simulink model "X31dynamics_03_controller_MG"  (R2014b)
settings: Solver=ode45  StartTime=0.0  StopTime=10.0  RelTol=1e-3
InitFcn:
  | X31dynamics_03_controller_MG_init
undefined symbols (not defined in the file or in its folder): X31_MnvrGen
libraries: simulink x10
settings Model: Creator=5909  LastModifiedBy=5909
settings OptimizationCC: InlineParams=on

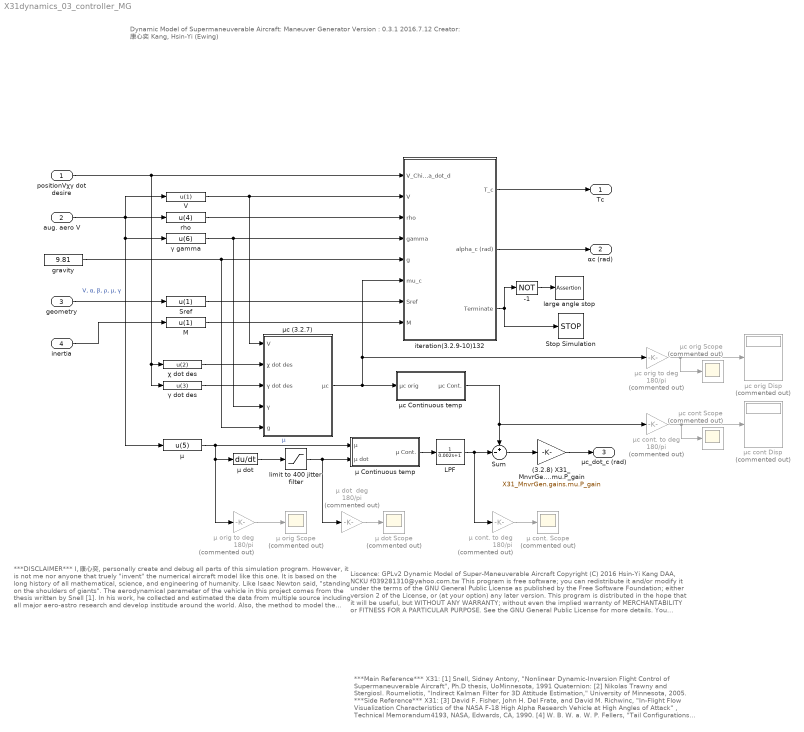
== system X31dynamics_03_controller_MG ==
  note: Dynamic Model of Supermaneuverable Aircraft:
      | Maneuver Generator
      | Version : 0.3.1
      | 2016.7.12
      | Creator: 康心奕 Kang, Hsin-Yi (Ewing)
  note: Liscence: GPLv2
      | Dynamic Model of Super-Maneuverable Aircraft
      | Copyright (C) 2016 Hsin-Yi Kang
      | DAA, NCKU
      | f039281310@yahoo.com.tw
      | This program is free software; you can redistribute it and/or modify it under the terms of the GNU General Public License as published by the Free Software Foundation; either version 2 of the License, or (at your option) any later version. This program is distributed in the hope that it will be useful, but WITHOUT ANY WARRANTY; without even the implied warranty of MERCHANTABILITY or FITNESS FOR A PARTICULAR PURPOSE. See the GNU General Public License for more details. You should have received a copy of the GNU General Public License along with this program; if not, write to the Free Software Foundation, Inc., 51 Franklin Street, Fifth Floor, Boston, MA 02110-1301, USA.
  note: ***DISCLAIMER***
      | I, 康心奕, personally create and debug all parts of this simulation program. However, it is not me nor anyone that truely "invent" the numerical aircraft model like this one. It is based on the long history of all mathematical, science, and engineering of humanity. Like Isaac Newton said, "standing on the shoulders of giants".
      | The aerodynamical parameter of the vehicle in this project comes from the thesis written by Snell [1]. In his work, he collected and estimated the data from multiple source including all major aero-astro research and develop institude around the world. Also, the method to model the dynamics of the vehicle and the controller implemented including the NDI and Gain Scheduling also came from his thesis.
      | The quaternion kinematics mainly reference to the toturial paper done by Trawny [2], where he collected and organized all fundamental properties and mathematical operation of such system.
      | This model is released to improve our ability to understand and develop control methodology of aerial vehicle system similar to this one. It is released free of charge now and always will be so in the hope of sharing the knowledge as much as possible and making this world a better place.
      | However, despite my greatest effort to ensure the correctness of the code, it is not garantee to be free of bug or other issue. You are free to use and modify the program to meet your need but I'm not responsible for any potential risk or damaged of any kind.
      |
      | Long live and prosper
  note: ***Main Reference***
      | X31:
      | [1] Snell, Sidney Antony, "Nonlinear Dynamic-Inversion Flight Control of Supermaneuverable Aircraft", Ph.D thesis, UoMinnesota, 1991
      | Quaternion:
      | [2] Nikolas Trawny and StergiosI. Roumeliotis, "Indirect Kalman Filter for 3D Attitude Estimation," University of Minnesota, 2005.
      |
      | ***Side Reference***
      | X31:
      | [3] David F. Fisher, John H. Del Frate, and David M. Richwinc, "In-Flight Flow Visualization Characteristics of the NASA F-18 High Alpha Research Vehicle at High Angles of Attack"
      | , Technical Memorandum4193, NASA, Edwards, CA, 1990.
      | [4] W. B. W. a. W. P. Fellers, "Tail Configurations for Highly Maneuverable Aircraft," AGARD, 1981.
      |
      | Quaternion:
      | [5] Nikolas Trawnyand StergiosI. Roumeliotis, "Indirect Kalman Filter for 3D Attitude Estimation," University of Minnesota, 2005.
      | [6] W. G. Breckenridge, "Quaternions -Proposed Standard Conventions," JPL, Tech. Rep. INTEROFFICE MEMORANDUM 343-79-1199, 1999.
      | [7] D. M. Henderson, "EularAngles, Quaternions, and Transformation Matrices," Mission Planning and Analysis Division, NASA, July 1977.
  positionVχγ dot desire : Inport  PortDimensions=3
  aug. aero V : Inport  Port=2  PortDimensions=6
  geometry : Inport  Port=3  PortDimensions=7
  inertia : Inport  Port=4  PortDimensions=7
  (3.2.8) X31_MnvrGen.gains.mu.P_gain : Gain  Gain=X31_MnvrGen.gains.mu.P_gain
  -1 : Logic  Operator=NOT  AllPortsSameDT=off  OutDataTypeStr=boolean
  LPF : TransferFcn  Denominator=[0.002 1]
  M : Fcn  Expr=u(1)
  Sref : Fcn  Expr=u(1)
  Stop Simulation : Stop
  Sum : Sum  Inputs=+-|
  V : Fcn  Expr=u(1)
  gravity : Constant  Value=9.81
  iteration(3.2.9-10)132 : Subsystem
  large angle stop : Assertion  AssertionFailFcn=warning('Maneuver Generator fails with large angle')  StopWhenAssertionFail=off
  limit to 400 jitter filter : Saturate  UpperLimit=400  LowerLimit=-400
  rho : Fcn  Expr=u(4)
  γ dot des : Fcn  Expr=u(3)
  γ gamma : Fcn  Expr=u(6)
  μ : Fcn  Expr=u(5)
  μ Continuous temp : Subsystem
  μ cont. Scope : Scope  Commented=on
      settings: YMin=-400  YMax=0  SaveName=ScopeData21
  μ cont. to deg : Gain  Commented=on  Gain=180/pi
  μ dot : Derivative
  μ dot  deg : Gain  Commented=on  Gain=180/pi
  μ dot Scope : Scope  Commented=on
      settings: YMin=-3e+08  YMax=1e+08  SaveName=ScopeData2
  μ orig Scope : Scope  Commented=on
      settings: YMin=-200  YMax=100
  μ orig to deg : Gain  Commented=on  Gain=180/pi
  μc (3.2.7) : Subsystem
  μc Continuous temp : Subsystem
  μc cont Disp : Display  Commented=on
  μc cont Scope : Scope  Commented=on
      settings: TimeRange=3.005065038857998  YMin=-240  YMax=-195
  μc cont. to deg : Gain  Commented=on  Gain=180/pi
  μc orig Disp : Display  Commented=on
  μc orig Scope : Scope  Commented=on
      settings: TimeRange=3.005065038857998  YMin=-200  YMax=200  SaveName=ScopeData14
  μc orig to deg : Gain  Commented=on  Gain=180/pi
  χ dot des : Fcn  Expr=u(2)
  Tc : Outport  PortDimensions=1
  αc (rad) : Outport  Port=2  PortDimensions=1
  μc_dot_c (rad) : Outport  Port=3  PortDimensions=1
  wires:
  positionVχγ dot desire/1 -> γ dot des/1, χ dot des/1, iteration(3.2.9-10)132/1(V_Chi_Gamma_dot_d)
  aug. aero V/1 -> μ/1, γ gamma/1, V/1, rho/1  "V, α, β, ρ, μ, γ"
  Sum/1 -> (3.2.8) X31_MnvrGen.gains.mu.P_gain/1
  (3.2.8) X31_MnvrGen.gains.mu.P_gain/1 -> μc_dot_c (rad)/1
  iteration(3.2.9-10)132/2(alpha_c (rad)) -> αc (rad)/1
  iteration(3.2.9-10)132/1(T_c) -> Tc/1
  geometry/1 -> Sref/1
  inertia/1 -> M/1
  V/1 -> μc (3.2.7)/1(V), iteration(3.2.9-10)132/2(V)
  γ dot des/1 -> μc (3.2.7)/3(γ dot des)
  χ dot des/1 -> μc (3.2.7)/2(χ dot des)
  gravity/1 -> μc (3.2.7)/5(g), iteration(3.2.9-10)132/5(g)
  γ gamma/1 -> μc (3.2.7)/4(γ), iteration(3.2.9-10)132/4(gamma)
  rho/1 -> iteration(3.2.9-10)132/3(rho)
  iteration(3.2.9-10)132/3(Terminate) -> Stop Simulation/1, -1/1
  Sref/1 -> iteration(3.2.9-10)132/7(Sref)
  M/1 -> iteration(3.2.9-10)132/8(M)
  -1/1 -> large angle stop/1
  μ cont. to deg/1 -> μ cont. Scope/1
  μ dot/1 -> limit to 400 jitter filter/1
  μc (3.2.7)/1(μc) -> iteration(3.2.9-10)132/6(mu_c), μc orig to deg/1, μc Continuous temp/1(μc orig)
  μ orig to deg/1 -> μ orig Scope/1
  μ/1 -> μ Continuous temp/1(μ), μ dot/1, μ orig to deg/1  "μ"
  μc orig to deg/1 -> μc orig Disp/1, μc orig Scope/1
  μc Continuous temp/1("μc Cont. ") -> μc cont. to deg/1, Sum/1
  μc cont. to deg/1 -> μc cont Disp/1, μc cont Scope/1
  μ dot  deg/1 -> μ dot Scope/1
  μ Continuous temp/1(μ Cont.) -> LPF/1
  LPF/1 -> Sum/2, μ cont. to deg/1
  limit to 400 jitter filter/1 -> μ Continuous temp/2(μ dot), μ dot  deg/1

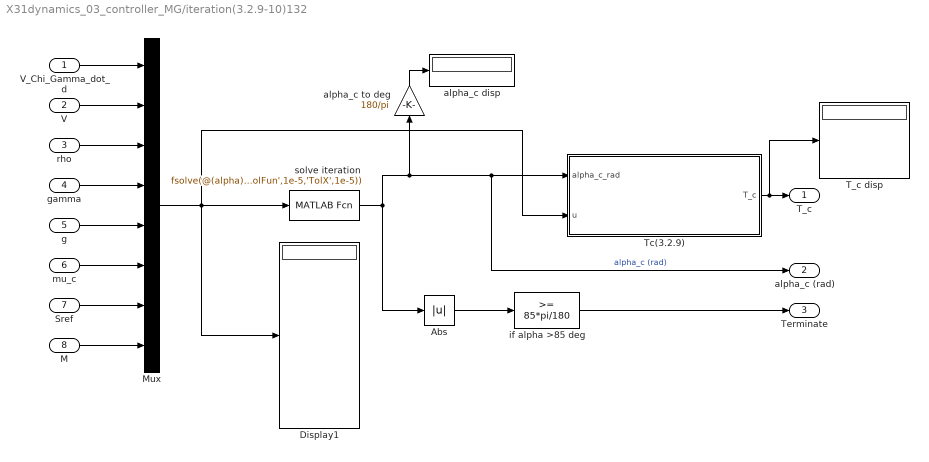
== system X31dynamics_03_controller_MG/iteration(3.2.9-10)132 ==
  V_Chi_Gamma_dot_d : Inport
  V : Inport  Port=2
  rho : Inport  Port=3
  gamma : Inport  Port=4
  g : Inport  Port=5
  mu_c : Inport  Port=6
  Sref : Inport  Port=7
  M : Inport  Port=8
  Abs : Abs
  Display1 : Display
  Mux : Mux  Inputs=8
  T_c disp : Display
  Tc(3.2.9) : MATLAB Function  TreatAsAtomicUnit=on
  alpha_c disp : Display
  alpha_c to deg : Gain  Gain=180/pi
  if alpha >85 deg : simulink/Logic and Bit Operations/Compare To Constant  relop=>=  const=85*pi/180  OutDataTypeStr=boolean
  solve iteration : MATLABFcn  MATLABFcn="fsolve(@(alpha)X31dynamics_03_controller_MG_iter_3_2_9_10(alpha, u(1),u(2), u(3), u(4), u(5),u(6), u(7), u(8), u(9), u(10) ),  10*pi/180, optimset('Display','off', 'TolFun',1e-5,'TolX',1e-5))"
  T_c : Outport
  alpha_c (rad) : Outport  Port=2
  Terminate : Outport  Port=3
  wires:
  V_Chi_Gamma_dot_d/1 -> Mux/1
  V/1 -> Mux/2
  rho/1 -> Mux/3
  gamma/1 -> Mux/4
  g/1 -> Mux/5
  mu_c/1 -> Mux/6
  Sref/1 -> Mux/7
  M/1 -> Mux/8
  Mux/1 -> Display1/1, solve iteration/1, Tc(3.2.9)/2(u)
  solve iteration/1 -> alpha_c (rad)/1, Tc(3.2.9)/1(alpha_c_rad), alpha_c to deg/1, Abs/1  "alpha_c (rad)"
  if alpha >85 deg/1 -> Terminate/1
  Tc(3.2.9)/1(T_c) -> T_c disp/1, T_c/1
  Abs/1 -> if alpha >85 deg/1
  alpha_c to deg/1 -> alpha_c disp/1

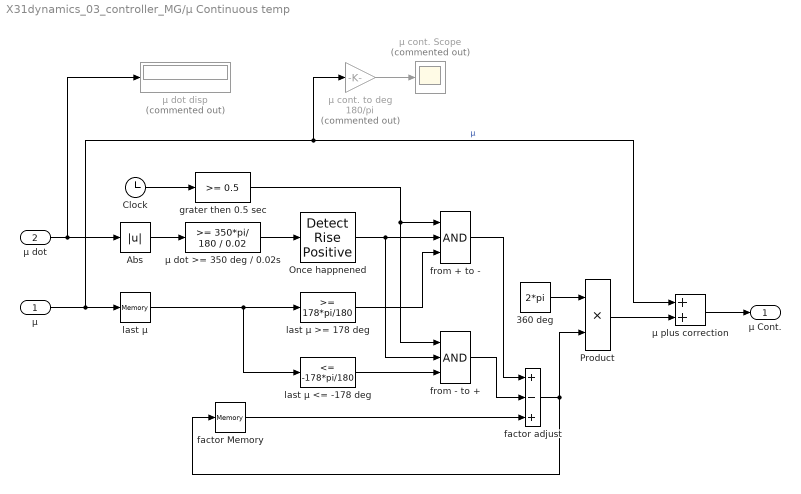
== system X31dynamics_03_controller_MG/μ Continuous temp ==
  μ : Inport
  μ dot : Inport  Port=2
  360 deg : Constant  Value=2*pi
  Abs : Abs
  Clock : Clock
  Once happnened : simulink/Logic and Bit Operations/Detect Rise Positive  vinit=0  InputProcessing=Inherited  OutDataTypeStr=boolean
  Product : Product
  factor Memory : Memory
  factor adjust : Sum  Inputs=+-+
  from + to - : Logic  Inputs=3  AllPortsSameDT=off  OutDataTypeStr=fixdt(1,16)
  from - to + : Logic  Inputs=3  AllPortsSameDT=off  OutDataTypeStr=fixdt(1,16)
  grater then 0.5 sec : simulink/Logic and Bit Operations/Compare To Constant  relop=>=  const=0.5  OutDataTypeStr=boolean
  last μ : Memory
  last μ <= -178 deg : simulink/Logic and Bit Operations/Compare To Constant  relop=<=  const=-178*pi/180  OutDataTypeStr=boolean
  last μ >= 178 deg : simulink/Logic and Bit Operations/Compare To Constant  relop=>=  const=178*pi/180  OutDataTypeStr=boolean
  μ cont. Scope : Scope  Commented=on
      settings: YMin=-200  YMax=200  SaveName=ScopeData3
  μ cont. to deg : Gain  Commented=on  Gain=180/pi
  μ dot >= 350 deg / 0.02s : simulink/Logic and Bit Operations/Compare To Constant  relop=>=  const=350*pi/ 180 / 0.02  OutDataTypeStr=uint8
  μ dot disp : Display  Commented=on
  μ plus correction : Sum
  μ Cont. : Outport  LibraryBlock=mblibv1/Utilities/Continuous Angle/Continuous Angle
  wires:
  μ dot/1 -> Abs/1, μ dot disp/1
  Abs/1 -> μ dot >= 350 deg / 0.02s/1
  last μ >= 178 deg/1 -> from + to -/3
  Once happnened/1 -> from + to -/2, from - to +/2
  factor adjust/1 -> factor Memory/1, Product/2
  factor Memory/1 -> factor adjust/3
  from + to -/1 -> factor adjust/1
  μ plus correction/1 -> μ Cont./1
  360 deg/1 -> Product/1
  Product/1 -> μ plus correction/2
  μ dot >= 350 deg / 0.02s/1 -> Once happnened/1
  last μ/1 -> last μ <= -178 deg/1, last μ >= 178 deg/1
  grater then 0.5 sec/1 -> from - to +/1, from + to -/1
  Clock/1 -> grater then 0.5 sec/1
  μ cont. to deg/1 -> μ cont. Scope/1
  μ/1 -> μ plus correction/1, μ cont. to deg/1, last μ/1  "μ"
  last μ <= -178 deg/1 -> from - to +/3
  from - to +/1 -> factor adjust/2

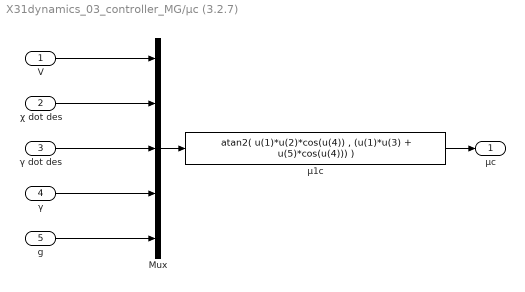
== system X31dynamics_03_controller_MG/μc (3.2.7) ==
  V : Inport
  χ dot des : Inport  Port=2
  γ dot des : Inport  Port=3
  γ : Inport  Port=4
  g : Inport  Port=5
  Mux : Mux  Inputs=5
  μ1c : Fcn  Expr="atan2(  u(1)*u(2)*cos(u(4)) , (u(1)*u(3) + u(5)*cos(u(4)))  )"
  μc : Outport
  wires:
  V/1 -> Mux/1
  χ dot des/1 -> Mux/2
  γ dot des/1 -> Mux/3
  g/1 -> Mux/5
  Mux/1 -> μ1c/1
  μ1c/1 -> μc/1
  γ/1 -> Mux/4

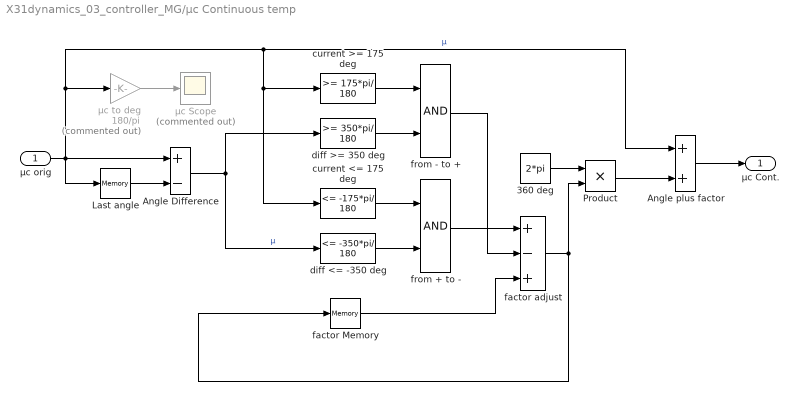
== system X31dynamics_03_controller_MG/μc Continuous temp ==
  μc orig : Inport
  360 deg : Constant  Value=2*pi
  Angle Difference : Sum  Inputs=+-
  Angle plus factor : Sum
  Last angle : Memory
  Product : Product
  current <= 175 deg : simulink/Logic and Bit Operations/Compare To Constant  relop=<=  const=-175*pi/ 180  OutDataTypeStr=boolean
  current >= 175 deg : simulink/Logic and Bit Operations/Compare To Constant  relop=>=  const=175*pi/ 180  OutDataTypeStr=boolean
  diff <= -350 deg : simulink/Logic and Bit Operations/Compare To Constant  relop=<=  const=-350*pi/ 180  OutDataTypeStr=boolean
  diff >= 350 deg : simulink/Logic and Bit Operations/Compare To Constant  relop=>=  const=350*pi/ 180  OutDataTypeStr=boolean
  factor Memory : Memory
  factor adjust : Sum  Inputs=+-+
  from + to - : Logic  AllPortsSameDT=off  OutDataTypeStr=fixdt(1,16)
  from - to + : Logic  AllPortsSameDT=off  OutDataTypeStr=fixdt(1,16)
  μc Scope : Scope  Commented=on
      settings: YMin=-200  YMax=200  SaveName=ScopeData4
  μc to deg : Gain  Commented=on  Gain=180/pi
  "μc Cont. " : Outport  LibraryBlock=mblibv1/Utilities/Continuous Angle/Continuous Angle
  wires:
  diff >= 350 deg/1 -> from - to +/2
  current >= 175 deg/1 -> from - to +/1
  factor adjust/1 -> factor Memory/1, Product/2
  factor Memory/1 -> factor adjust/3
  from - to +/1 -> factor adjust/2
  Angle plus factor/1 -> "μc Cont. "/1
  Last angle/1 -> Angle Difference/2
  360 deg/1 -> Product/1
  Product/1 -> Angle plus factor/2
  diff <= -350 deg/1 -> from + to -/2
  from + to -/1 -> factor adjust/1
  μc to deg/1 -> μc Scope/1
  μc orig/1 -> μc to deg/1, Angle plus factor/1, current <= 175 deg/1, current >= 175 deg/1, Last angle/1, Angle Difference/1  "μ"
  Angle Difference/1 -> diff <= -350 deg/1, diff >= 350 deg/1  "μ"
  current <= 175 deg/1 -> from + to -/1

== matlab function X31dynamics_03_controller_MG/iteration(3.2.9-10)132/Tc(3.2.9) ==
  data: alpha_c_rad input; u input; T_c output; X31_MnvrGen parameter
function T_c = Tc_from_alpha_C(alpha_c_rad, u, X31_MnvrGen)
V_dot_d = u(1);
V = u(4);
rho = u(5);
gamma = u(6);
g = u(7);
Sref = u(9);
M = u(10);

% Drag
alpha_c_deg = 180 / pi * alpha_c_rad;   % convert to degree for polynomials
a_abs = abs(alpha_c_deg);

fig2_2_1b = X31_MnvrGen.aero_poly.fig2_2(1).b;
      % figer 2.2.1b is the Drag coefficient
CD = fig2_2_1b(6)*a_abs^6 + fig2_2_1b(5)*a_abs^5 + fig2_2_1b(4)*a_abs^4 +...
                fig2_2_1b(3)*a_abs^3 + fig2_2_1b(2)*a_abs^2 + fig2_2_1b(1)*a_abs + fig2_2_1b(7);
Drag = 0.5*rho*V^2*Sref*CD;

T_c = 1/cos(alpha_c_rad) * (M*V_dot_d + Drag + M*g*sin(gamma));
end
